simulink model "GantryCrane"  (R2017a)
settings: Solver=ode4  StartTime=0.0  StopTime=10  FixedStep=0.1  RelTol=1e-3
InitFcn:
  | Crane_Data
values from neighbouring files (symbols this model uses):
  g = 9.81    [Crane_Data.m]    (also in initMIMOgpc.m = mat2cell(gaux,n,m*ones(1,N2)))
  l = 0.5    [Crane_Data.m]
  m1 = 0.5    [Crane_Data.m]
  m2 = 2    [Crane_Data.m]
libraries: simulink x2
settings Model: Creator=Daniel  LastModifiedBy=Daniel

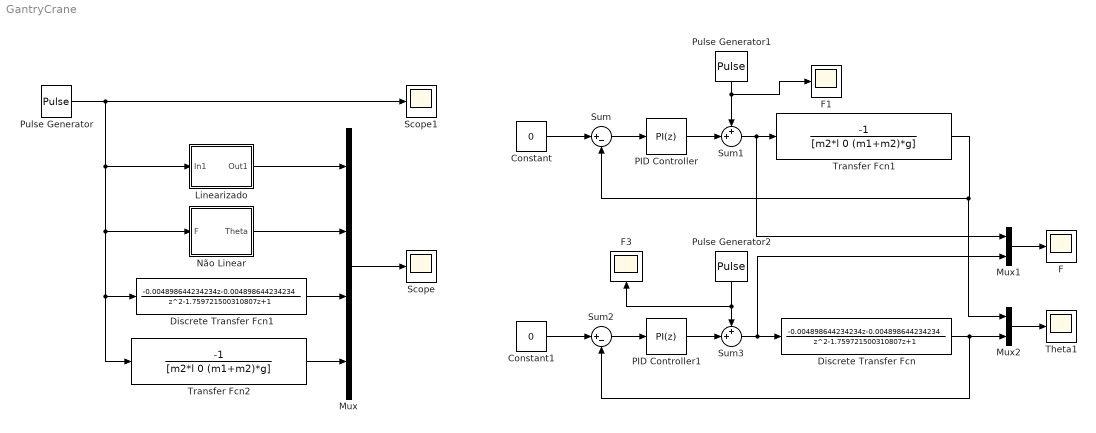
== system GantryCrane ==
  Constant : Constant  Value=0
  Constant1 : Constant  Value=0
  Discrete Transfer Fcn : DiscreteTransferFcn  Numerator="[-0.004898644234234  -0.004898644234234]"  Denominator=[1 -1.759721500310807 1]
  Discrete Transfer Fcn1 : DiscreteTransferFcn  Numerator="[-0.004898644234234  -0.004898644234234]"  Denominator=[1 -1.759721500310807 1]
  F : Scope
  F1 : Scope
  F3 : Scope
  Linearizado : Subsystem
  Mux : Mux
  Mux1 : Mux  Inputs=2
  Mux2 : Mux  Inputs=2
  Não Linear : Subsystem
  PID Controller : simulink/Continuous/PID Controller  Controller=PI  TimeDomain=Discrete-time  SampleTime=-1  IntegratorMethod=Forward Euler  FilterMethod=Forward Euler  Form=Parallel  UseFilter=on  ControllerParametersSource=internal  P=-200  I=-100  D=0  N=100  InitialConditionSource=internal  InitialConditionForIntegrator=0  InitialConditionForFilter=0  ExternalReset=none  LimitOutput=off  UpperSaturationLimit=inf  LowerSaturationLimit=-inf  LinearizeAsGain=on  AntiWindupMode=none  Kb=1  TrackingMode=off  Kt=1  PParamMin=[]  PParamMax=[]  IParamMin=[]  IParamMax=[]  DParamMin=[]  DParamMax=[]  NParamMin=[]  NParamMax=[]  KbParamMin=[]  KbParamMax=[]  KtParamMin=[]  KtParamMax=[]  POutMin=[]  POutMax=[]  IOutMin=[]  IOutMax=[]  DOutMin=[]  DOutMax=[]  NOutMin=[]  NOutMax=[]  KbOutMin=[]  KbOutMax=[]  KtOutMin=[]  KtOutMax=[]  IntegratorOutMin=[]  IntegratorOutMax=[]  FilterOutMin=[]  FilterOutMax=[]  SumOutMin=[]  SumOutMax=[]  SumI1OutMin=[]  SumI1OutMax=[]  SumI2OutMin=[]  SumI2OutMax=[]  SumI3OutMin=[]  SumI3OutMax=[]  SumDOutMin=[]  SumDOutMax=[]  SaturationOutMin=[]  SaturationOutMax=[]  IntegratorContinuousStateAttributes=''  IntegratorStateMustResolveToSignalObject=off  IntegratorRTWStateStorageClass=Auto  FilterContinuousStateAttributes=''  FilterStateMustResolveToSignalObject=off  FilterRTWStateStorageClass=Auto  DifferentiatorICPrevScaledInput=0  DifferentiatorOutMin=[]  DifferentiatorOutMax=[]  InitialConditionSetting=State (most efficient)
  PID Controller1 : simulink/Continuous/PID Controller  Controller=PI  TimeDomain=Discrete-time  SampleTime=-1  IntegratorMethod=Forward Euler  FilterMethod=Forward Euler  Form=Parallel  UseFilter=on  ControllerParametersSource=internal  P=-1  I=-1  D=1  N=100  InitialConditionSource=internal  InitialConditionForIntegrator=0  InitialConditionForFilter=0  ExternalReset=none  LimitOutput=off  UpperSaturationLimit=inf  LowerSaturationLimit=-inf  LinearizeAsGain=on  AntiWindupMode=none  Kb=1  TrackingMode=off  Kt=1  PParamMin=[]  PParamMax=[]  IParamMin=[]  IParamMax=[]  DParamMin=[]  DParamMax=[]  NParamMin=[]  NParamMax=[]  KbParamMin=[]  KbParamMax=[]  KtParamMin=[]  KtParamMax=[]  POutMin=[]  POutMax=[]  IOutMin=[]  IOutMax=[]  DOutMin=[]  DOutMax=[]  NOutMin=[]  NOutMax=[]  KbOutMin=[]  KbOutMax=[]  KtOutMin=[]  KtOutMax=[]  IntegratorOutMin=[]  IntegratorOutMax=[]  FilterOutMin=[]  FilterOutMax=[]  SumOutMin=[]  SumOutMax=[]  SumI1OutMin=[]  SumI1OutMax=[]  SumI2OutMin=[]  SumI2OutMax=[]  SumI3OutMin=[]  SumI3OutMax=[]  SumDOutMin=[]  SumDOutMax=[]  SaturationOutMin=[]  SaturationOutMax=[]  IntegratorContinuousStateAttributes=''  IntegratorStateMustResolveToSignalObject=off  IntegratorRTWStateStorageClass=Auto  FilterContinuousStateAttributes=''  FilterStateMustResolveToSignalObject=off  FilterRTWStateStorageClass=Auto  DifferentiatorICPrevScaledInput=0  DifferentiatorOutMin=[]  DifferentiatorOutMax=[]  InitialConditionSetting=State (most efficient)
  Pulse Generator : DiscretePulseGenerator  PulseType=Time based  Period=20  PulseWidth=5
  Pulse Generator1 : DiscretePulseGenerator  PulseType=Time based  Period=20  PulseWidth=5
  Pulse Generator2 : DiscretePulseGenerator  PulseType=Time based  Period=20  PulseWidth=5
  Scope : Scope
  Scope1 : Scope
  Sum : Sum  Inputs=|+-
  Sum1 : Sum  Inputs=++|
  Sum2 : Sum  Inputs=|+-
  Sum3 : Sum  Inputs=++|
  Theta1 : Scope
  Transfer Fcn1 : TransferFcn  Numerator=[-1]  Denominator=[m2*l 0 (m1+m2)*g]
  Transfer Fcn2 : TransferFcn  Numerator=[-1]  Denominator=[m2*l 0 (m1+m2)*g]
  wires:
  Mux/1 -> Scope/1
  Não Linear/1(Theta) -> Mux/2
  Linearizado/1(Out1) -> Mux/1
  Pulse Generator/1 -> Scope1/1, Linearizado/1(In1), Discrete Transfer Fcn1/1, Transfer Fcn2/1, Não Linear/1(F)
  Transfer Fcn1/1 -> Mux2/1, Sum/2
  Constant/1 -> Sum/1
  Pulse Generator1/1 -> F1/1, Sum1/1
  Sum/1 -> PID Controller/1
  Sum1/1 -> Mux1/1, Transfer Fcn1/1
  Mux2/1 -> Theta1/1
  Sum2/1 -> PID Controller1/1
  Pulse Generator2/1 -> F3/1, Sum3/1
  Constant1/1 -> Sum2/1
  Discrete Transfer Fcn/1 -> Mux2/2, Sum2/2
  Sum3/1 -> Mux1/2, Discrete Transfer Fcn/1
  Transfer Fcn2/1 -> Mux/4
  Mux1/1 -> F/1
  PID Controller/1 -> Sum1/2
  PID Controller1/1 -> Sum3/2
  Discrete Transfer Fcn1/1 -> Mux/3

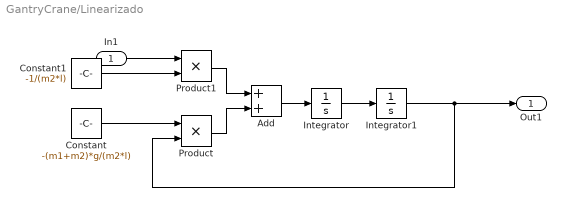
== system GantryCrane/Linearizado ==
  In1 : Inport
  Add : Sum
  Constant : Constant  Value=-(m1+m2)*g/(m2*l)
  Constant1 : Constant  Value=-1/(m2*l)
  Integrator : Integrator
  Integrator1 : Integrator
  Product : Product
  Product1 : Product
  Out1 : Outport
  wires:
  Integrator/1 -> Integrator1/1
  Constant/1 -> Product/1
  Integrator1/1 -> Product/2, Out1/1
  Add/1 -> Integrator/1
  Constant1/1 -> Product1/2
  Product/1 -> Add/2
  Product1/1 -> Add/1
  In1/1 -> Product1/1

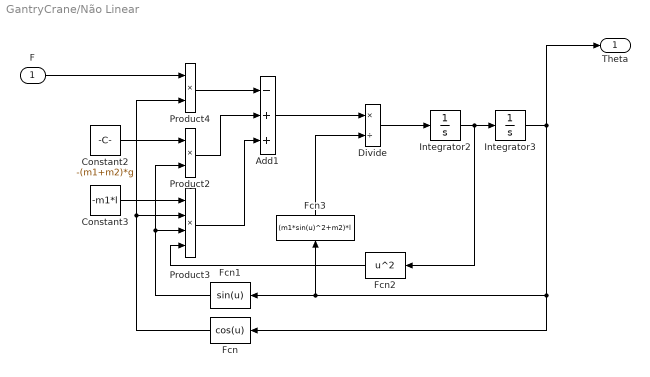
== system GantryCrane/Não Linear ==
  F : Inport
  Add1 : Sum  Inputs=-++
  Constant2 : Constant  Value=-(m1+m2)*g
  Constant3 : Constant  Value=-m1*l
  Divide : Product  Inputs=*/
  Fcn : Fcn  Expr=cos(u)
  Fcn1 : Fcn  Expr=sin(u)
  Fcn2 : Fcn  Expr=u^2
  Fcn3 : Fcn  Expr=(m1*sin(u)^2+m2)*l
  Integrator2 : Integrator
  Integrator3 : Integrator
  Product2 : Product
  Product3 : Product  Inputs=4
  Product4 : Product
  Theta : Outport
  wires:
  Add1/1 -> Divide/1
  Product3/1 -> Add1/3
  Integrator3/1 -> Theta/1, Fcn/1, Fcn3/1, Fcn1/1
  Integrator2/1 -> Fcn2/1, Integrator3/1
  Fcn2/1 -> Product3/4
  Constant2/1 -> Product2/1
  Product4/1 -> Add1/1
  Divide/1 -> Integrator2/1
  Fcn1/1 -> Product2/2, Product3/3
  Fcn/1 -> Product4/2, Product3/2
  Product2/1 -> Add1/2
  Constant3/1 -> Product3/1
  Fcn3/1 -> Divide/2
  F/1 -> Product4/1
